simulink model "wcb2"  (R2024b)
settings: Solver=VariableStepAuto  StartTime=0.0  StopTime=10.0  RelTol=1e-3
undefined symbols (not defined in the file): doppler
libraries: commchan3 x2, simulink x2, commdigbbndpm3 x2, commsink2 x1, commrandsrc3 x1
settings Model: Creator=anaht  LastModifiedBy=anaht

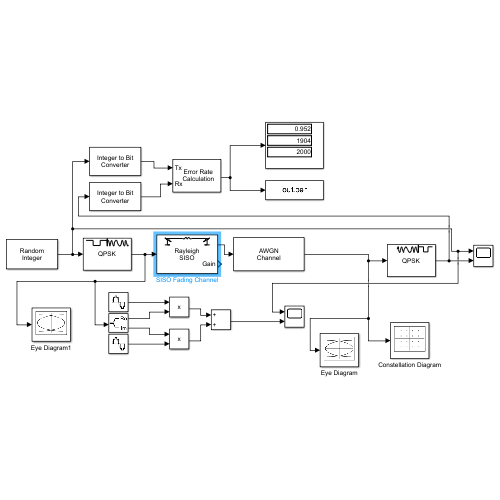
[thumbnail: Simulink's stored preview of the top-level diagram]
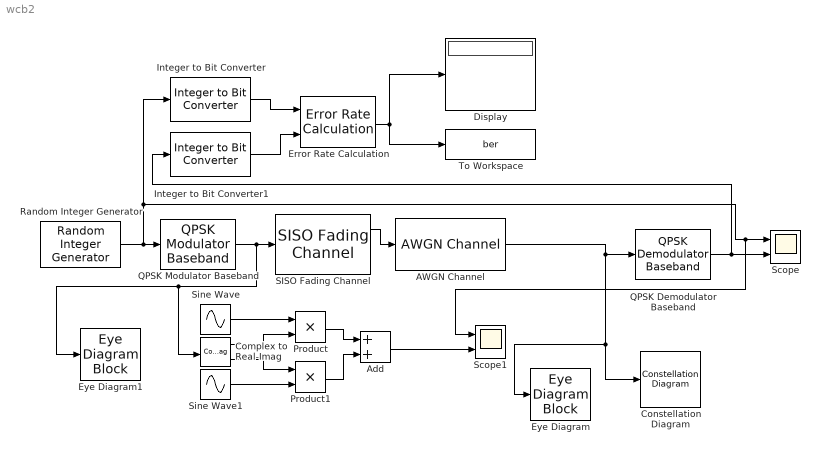
== system wcb2 ==
  AWGN Channel : commchan3/AWGN Channel  LegacyMode=off  NoiseMethod="Signal to noise ratio  (Eb/No)"  noiseMode="Signal to noise ratio  (SNR)"  EbNo=20  EsNo=10  SNR=10  BitsPerSymbol=2  SignalPower=1  SamplesPerSymbol=1  SymbolPeriod=1  VarianceSource=Parameter  Variance=1  RandomStream=Global stream  Seed=67  SimulateUsing=Code generation
  Add : Sum
  Complex to Real-Imag : ComplexToRealImag
  Constellation Diagram : ConstellationDiagram  WindowPosition=[340.000000,60.000000,600.000000,600.000000,]  Visible=on  ScopeFrameLocation=window
  Display : Display
  Error Rate Calculation : commsink2/Error Rate Calculation  N=0  st_delay=0  cp_mode=Entire frame  subframe=[]  PMode=Port  WsName=ErrorVec  RsMode2=off  stop=off  numErr=100  maxBits=1e6
  Eye Diagram : EyeDiagramBlock  WindowPosition=[240.000000,110.000000,800.000000,500.000000,]  ScopeFrameLocation=window  SamplesPerSymbol=1  YLimits=[-1.1,1.1]
  Eye Diagram1 : EyeDiagramBlock  WindowPosition=[240.000000,110.000000,800.000000,500.000000,]  ScopeFrameLocation=window  SamplesPerSymbol=1  YLimits=[-1.1,1.1]
  Integer to Bit Converter : simulink/Logic and Bit Operations/Integer to Bit Converter  nbits=2  signedInputValues=Unsigned  bitOrder=MSB first  outDtype=Inherit via internal rule
  Integer to Bit Converter1 : simulink/Logic and Bit Operations/Integer to Bit Converter  nbits=2  signedInputValues=Unsigned  bitOrder=MSB first  outDtype=Inherit via internal rule
  Product : Product
  Product1 : Product
  QPSK Demodulator Baseband : commdigbbndpm3/QPSK Demodulator Baseband  OutType=Integer  DecType=Hard decision  VarSource=Dialog  Variance=1  Dec=Gray  Ph=pi/4  outDtype1=Inherit via internal rule  outDtype2=Inherit via internal rule  derotateFactorWordLen=16  derotateFactorDataTypeStr=Inherit: Same word length as input  derotateFactorLastDataTypeStr=Inherit: Same word length as input
  QPSK Modulator Baseband : commdigbbndpm3/QPSK Modulator Baseband  InType=Integer  Enc=Gray  Ph=pi/4  outDtype=double  outWordLen=16  outUDDataType=sfix(16)  outFracLenMode=Best precision  outFracLen=15  outDataTypeStr=double  outLastDataTypeStr=double
  Random Integer Generator : commrandsrc3/Random Integer Generator  SetSize=4  SeedSource=Auto  Seed=0  SampleTime=1  SamplesPerFrame=1000  OutputDataType=double  SimulateUsing=Interpreted execution
  SISO Fading Channel : commchan3/SISO Fading Channel  InheritSampleRate=on  SampleRate=1  PathDelays=[1e-6 2e-6 5e-6]  AveragePathGains="[-10 -10  0]"  NormalizePathGains=on  FadingDistribution=Rayleigh  KFactor=3  DirectPathDopplerShift=0  DirectPathInitialPhase=0  MaximumDopplerShift=0.0001  DopplerSpectrum=doppler('Jakes')  RandomStream=mt19937ar with seed  Seed=73  PathGainsOutputPort=on  ChannelFilterDelayOutputPort=off  SimulateUsing=Interpreted execution  Visualization=Off  PathsForDopplerDisplay=1  SamplesToDisplay=25%
  Scope : Scope  NumInputPorts=2
  Scope1 : Scope  NumInputPorts=2
  Sine Wave : Sin  Frequency=pi*5  SampleTime=0.001
  Sine Wave1 : Sin  Frequency=pi*5  Phase=pi/2  SampleTime=0.001
  To Workspace : ToWorkspace  VariableName=ber  SampleTime=-1
      settings: Save2DSignal=2-D array (concatenate along first dimension)
  wires:
  Product/1 -> Add/1
  QPSK Modulator Baseband/1 -> Eye Diagram1/1, Complex to Real-Imag/1, SISO Fading Channel/1
  Complex to Real-Imag/2 -> Product1/1
  Sine Wave/1 -> Product/1
  Add/1 -> Scope1/2
  Integer to Bit Converter1/1 -> Error Rate Calculation/2
  Integer to Bit Converter/1 -> Error Rate Calculation/1
  Product1/1 -> Add/2
  Complex to Real-Imag/1 -> Product/2
  SISO Fading Channel/1 -> AWGN Channel/1
  Error Rate Calculation/1 -> To Workspace/1, Display/1
  Random Integer Generator/1 -> Integer to Bit Converter/1, Scope1/1, Scope/1, QPSK Modulator Baseband/1
  AWGN Channel/1 -> Constellation Diagram/1, Eye Diagram/1, QPSK Demodulator Baseband/1
  QPSK Demodulator Baseband/1 -> Integer to Bit Converter1/1, Scope/2
  Sine Wave1/1 -> Product1/2
